simulink model "AION_auto_control_realization"  (R2021a)
settings: configuration reference "AION_IDS_Speedgoat" (kept outside this file)
undefined symbols (not defined in the file): set_ADCU_info, set_lateral_control_info, set_longitudinal_control_info
settings Model: DataDictionary=AION_auto_control_realization.sldd  SimulationMode=external  Creator=Administrator  LastModifiedBy=Administrator
settings ConfigSetRef: SourceName=AION_IDS_Speedgoat

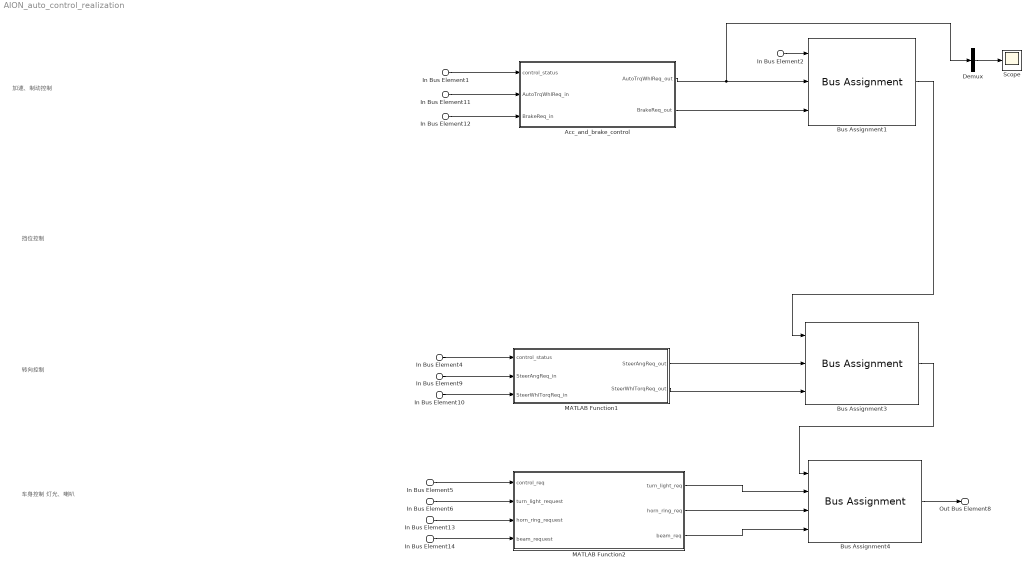
== system AION_auto_control_realization ==
  note: 加速、制动控制
  note: 挡位控制
  note: 转向控制
  note: 车身控制
      | 灯光、喇叭
  In Bus Element2 : Inport  PortName=InBus
  In Bus Element10 : Inport  PortName=InBus  Element=set_lateral_control_info.set_SteerWhlTorqReq
  In Bus Element9 : Inport  PortName=InBus  Element=set_lateral_control_info.set_SteerAngReq
  In Bus Element11 : Inport  PortName=InBus  Element=set_longitudinal_control_info.set_AutoTrqWhlReq
  In Bus Element12 : Inport  PortName=InBus  Element=set_longitudinal_control_info.set_BrakeReq
  In Bus Element14 : Inport  PortName=InBus  Element=set_ADCU_info.set_BeamReq
  In Bus Element5 : Inport  PortName=InBus  Element=set_ADCU_info.set_BodyCtrlReq
  In Bus Element13 : Inport  PortName=InBus  Element=set_ADCU_info.set_HornRingReq
  In Bus Element6 : Inport  PortName=InBus  Element=set_ADCU_info.set_TurnLightReq
  In Bus Element4 : Inport  PortName=InBus  Element=get_SCU_info.get_LatCtrlMode
  In Bus Element1 : Inport  PortName=InBus  Element=get_SCU_info.get_LngCtrlMode
  Acc_and_brake_control : MATLAB Function  TreatAsAtomicUnit=on
  Bus Assignment1 : BusAssignment  AssignedSignals=set_longitudinal_control_info.set_AutoTrqWhlReq,set_longitudinal_control_info.set_BrakeReq
  Bus Assignment3 : BusAssignment  AssignedSignals=set_lateral_control_info.set_SteerAngReq,set_lateral_control_info.set_SteerWhlTorqReq
  Bus Assignment4 : BusAssignment  AssignedSignals=set_ADCU_info.set_TurnLightReq,set_ADCU_info.set_HornRingReq,set_ADCU_info.set_BeamReq
  Demux : Demux  Outputs=1
  MATLAB Function1 : MATLAB Function  TreatAsAtomicUnit=on
  MATLAB Function2 : MATLAB Function  TreatAsAtomicUnit=on
  Scope : Scope
  Out Bus Element8 : Outport  PortName=OutBus
  wires:
  In Bus Element2/1 -> Bus Assignment1/1
  In Bus Element1/1 -> Acc_and_brake_control/1(control_status)
  In Bus Element4/1 -> MATLAB Function1/1(control_status)
  In Bus Element9/1 -> MATLAB Function1/2(SteerAngReq_in)
  In Bus Element10/1 -> MATLAB Function1/3(SteerWhlTorqReq_in)
  Bus Assignment1/1 -> Bus Assignment3/1
  MATLAB Function1/1(SteerAngReq_out) -> Bus Assignment3/2
  MATLAB Function1/2(SteerWhlTorqReq_out) -> Bus Assignment3/3
  In Bus Element12/1 -> Acc_and_brake_control/3(BrakeReq_in)
  Demux/1 -> Scope/1
  In Bus Element11/1 -> Acc_and_brake_control/2(AutoTrqWhlReq_in)
  Acc_and_brake_control/2(BrakeReq_out) -> Bus Assignment1/3
  Acc_and_brake_control/1(AutoTrqWhlReq_out) -> Bus Assignment1/2, Demux/1
  Bus Assignment3/1 -> Bus Assignment4/1
  In Bus Element5/1 -> MATLAB Function2/1(control_req)
  In Bus Element6/1 -> MATLAB Function2/2(turn_light_request)
  In Bus Element13/1 -> MATLAB Function2/3(horn_ring_request)
  In Bus Element14/1 -> MATLAB Function2/4(beam_request)
  MATLAB Function2/1(turn_light_req) -> Bus Assignment4/2
  MATLAB Function2/2(horn_ring_req) -> Bus Assignment4/3
  MATLAB Function2/3(beam_req) -> Bus Assignment4/4
  Bus Assignment4/1 -> Out Bus Element8/1

== matlab function AION_auto_control_realization/Acc_and_brake_control ==
  data: control_status input; AutoTrqWhlReq_out output uint32; AutoTrqWhlReq_in input; BrakeReq_in input; BrakeReq_out output
function [AutoTrqWhlReq_out,BrakeReq_out] = Acc_and_brake_control(control_status,AutoTrqWhlReq_in,BrakeReq_in)
%%
%输入参数
%AutoTrqWhlReq_in        轮端扭矩请求值
%BrakeReq_in             制动加速度请求值

%输出参数
%AutoTrqWhlReq_out      轮端扭矩输出值
%BrakeReq_out           制动加速度输出值
%%
% persistent BrakeReq_out 
% global AutoTrqWhlReq_out
% if isempty(BrakeReq_out)
%    BrakeReq_out = 0;
% end
% if isempty(AutoTrqWhlReq_out)
%    AutoTrqWhlReq_out = 0;
% end
%%
if(control_status == Control_status.AutoStatus )   
%只有在Auto状态下才能控制制动和加速
% %制动加速度控制
    if(BrakeReq_in > 0)
        BrakeReq_out = 0;
    elseif(BrakeReq_in < -10)
        BrakeReq_out = -10;
    else
        BrakeReq_out = BrakeReq_in;
    end
%同时存在加速和制动请求时，优先响应制动
    if(BrakeReq_in == 0)
        if(AutoTrqWhlReq_in < 0)
            AutoTrqWhlReq_out = 0;
        elseif(AutoTrqWhlReq_in  > 5000)
            AutoTrqWhlReq_out = 5000;
        else
            AutoTrqWhlReq_out = AutoTrqWhlReq_in;
        end
    else
        AutoTrqWhlReq_out = 0;
    end
else
    BrakeReq_out = 0;
    AutoTrqWhlReq_out = 0;
end
    AutoTrqWhlReq_out = AutoTrqWhlReq_out;
end
% function AutoTrqWhlReq_out = Acc_and_brake_control(control_status)
%  if(control_status == Control_status.AutoStatus )  
%      AutoTrqWhlReq_out = 50;
%  else
%      AutoTrqWhlReq_out = 30;
%  end
% end

== matlab function AION_auto_control_realization/MATLAB Function1 ==
  data: control_status input; SteerAngReq_out output; SteerAngReq_in input; SteerWhlTorqReq_in input; SteerWhlTorqReq_out output
function [SteerAngReq_out,SteerWhlTorqReq_out]= Steer_angle_control(control_status,SteerAngReq_in,SteerWhlTorqReq_in)
%%
%输入参数


%输出参数
%% 静态变量声明及初始化
% 初始化
persistent SteerWhlTorqReq_temp
if isempty(SteerWhlTorqReq_temp)
   SteerWhlTorqReq_temp = 0;
end
%%
if(control_status == Control_status.AutoStatus )   
%只有在Auto状态下才能控制转向
%请求转角范围为[-540,540],实际最大可执行角度为480
    if(SteerAngReq_in > 540)
        SteerAngReq_out = 540;
    elseif(SteerAngReq_in < -540)
        SteerAngReq_out = -540;
    else
        SteerAngReq_out = SteerAngReq_in;
    end
    
% 转向助力扭矩输出值计算，变化率不超过500deg/s，当前控制周期为0.02s  
%     if(SteerWhlTorqReq_in - SteerWhlTorqReq_temp > 10)
%         SteerWhlTorqReq_out = SteerWhlTorqReq_temp + 10;
%     elseif(SteerWhlTorqReq_in - SteerWhlTorqReq_temp < -10)
%         SteerWhlTorqReq_out = SteerWhlTorqReq_temp - 10;
%     else
%         SteerWhlTorqReq_out = SteerWhlTorqReq_in;
%     end
%     SteerWhlTorqReq_temp = SteerWhlTorqReq_out;
 
else
    SteerAngReq_out = 0;
end
    SteerWhlTorqReq_out = 0;
end

== matlab function AION_auto_control_realization/MATLAB Function2 ==
  data: control_req input; turn_light_req output; turn_light_request input; horn_ring_request input; beam_request input; horn_ring_req output; beam_req output
function [turn_light_req,horn_ring_req,beam_req] = body_control(control_req,...
    turn_light_request,horn_ring_request,beam_request)

%%
%初始话紧急灯计数变量
persistent EmergencyLightCount
if isempty(EmergencyLightCount)
    EmergencyLightCount = 0;
end
%%
if(control_req ==  Enable_request.Enable)
%车身控制请求处于激活指令，自动控制灯光、喇叭  
%1、转向灯请求   
%ADCU_TurnLightReq 必须先请求 NoRequset 再请求 Emergency light    
    if(turn_light_request == Light_request.EmergencyLight)
        if(EmergencyLightCount < 2)
        %TurnLightReq前2次发出EmergencyLight的指令，先请求No Request
            turn_light_req = Light_request.NoLightRequest ;
            EmergencyLightCount = EmergencyLightCount + 1;
        else
         %第3次发出EmergencyLight的指令，请求Emergency   
            turn_light_req = Light_request.EmergencyLight;
        end
    else
        %TurnLightReq发出左转或者右转的指令，直接按指令请求
         turn_light_req =  turn_light_request;
         EmergencyLightCount = 0;
    end
 %2、喇叭控制请求，直接响应指令   
    horn_ring_req = horn_ring_request;
 %3、大灯控制请求，直接响应指令
    beam_req = beam_request;
else
    turn_light_req = Light_request.NoLightRequest;
    horn_ring_req = Active_request.NotActiveRequest;
    beam_req = Beam_request.NoBeamRequest;
end
